simulink model "Kursach_kren"  (R2022b)
settings: Solver=VariableStepAuto  StartTime=0.0  StopTime=2  RelTol=1e-3
values from neighbouring files (symbols this model uses):
  k_omx = 1.2597    [obl_ust.m]
  k_sigm = 5.4231    [obl_ust.m]
  kzi_pr = sqrt(2)/2    [obl_ust.m]
  M_x_omx = -1    [obl_ust.m]
  M_x_sigme = -7    [obl_ust.m]
  om_pr = 20    [obl_ust.m]
libraries: checkpacklib x1
settings Model: Creator=79251  LastModifiedBy=79251

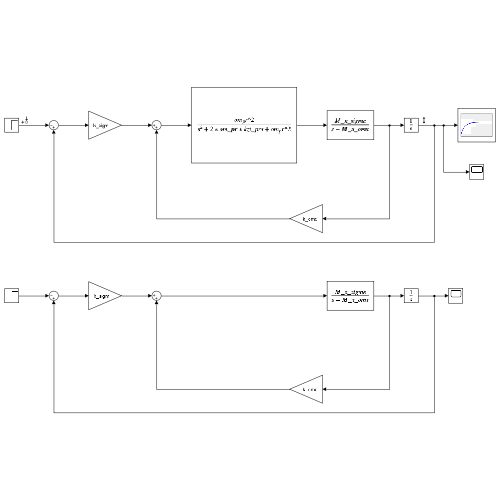
[thumbnail: Simulink's stored preview of the top-level diagram]
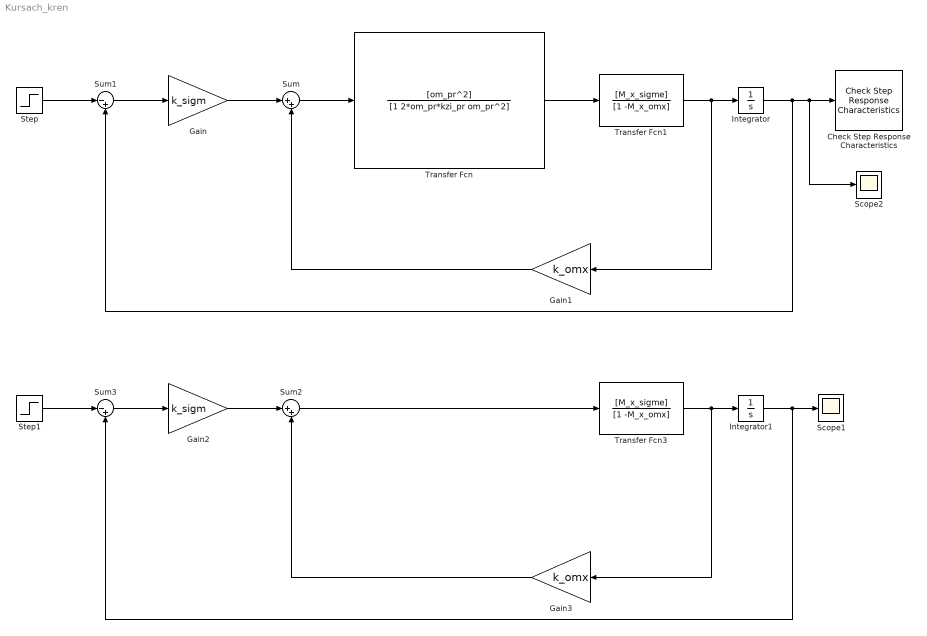
== system Kursach_kren ==
  Check Step Response Characteristics : checkpacklib/Check Step Response  Characteristics  InstantiateOnLoad=on  enabled=on  stopWhenAssertionFail=off  export=off  ViewDlgPos=[]  OpenViewOnLoad=off  LaunchViewOnOpen=off  TimeUnits=seconds  EnableStepResponseBound=on  InitialValue=0  FinalValue=1  StepTime=0  RiseTime=0.3  PercentRise=50  SettlingTime=0.4  PercentSettling=5  PercentOvershoot=5  PercentUndershoot=5
      settings: LibrarySourceBlock=|
      | sdolib/Model Verification/Check Step Response
      | Characteristics
  Gain : Gain  Gain=k_sigm
  Gain1 : Gain  Gain=k_omx
  Gain2 : Gain  Gain=k_sigm
  Gain3 : Gain  Gain=k_omx
  Integrator : Integrator
  Integrator1 : Integrator
  Scope1 : Scope
  Scope2 : Scope
  Step : Step  Time=0  SampleTime=0
  Step1 : Step  Time=0  SampleTime=0
  Sum : Sum  Inputs=|++
  Sum1 : Sum  Inputs=|-+
  Sum2 : Sum  Inputs=|++
  Sum3 : Sum  Inputs=|-+
  Transfer Fcn : TransferFcn  Numerator=[om_pr^2]  Denominator=[1 2*om_pr*kzi_pr om_pr^2]
  Transfer Fcn1 : TransferFcn  Numerator=[M_x_sigme]  Denominator=[1 -M_x_omx]
  Transfer Fcn3 : TransferFcn  Numerator=[M_x_sigme]  Denominator=[1 -M_x_omx]
  wires:
  Sum1/1 -> Gain/1
  Gain/1 -> Sum/1
  Step/1 -> Sum1/1
  Sum/1 -> Transfer Fcn/1
  Transfer Fcn/1 -> Transfer Fcn1/1
  Transfer Fcn1/1 -> Gain1/1, Integrator/1
  Gain1/1 -> Sum/2
  Transfer Fcn3/1 -> Gain3/1, Integrator1/1
  Sum2/1 -> Transfer Fcn3/1
  Gain3/1 -> Sum2/2
  Sum3/1 -> Gain2/1
  Integrator1/1 -> Sum3/2, Scope1/1
  Gain2/1 -> Sum2/1
  Step1/1 -> Sum3/1
  Integrator/1 -> Scope2/1, Check Step Response Characteristics/1, Sum1/2
